simulink library "plant_sim_lib"  (R2022b)
settings: Solver=VariableStepAuto  StartTime=0.0  StopTime=10.0  RelTol=1e-3
libraries: AMK_model_lib x1, battery_model_lib x1, driver_model_lib x1
settings Model: Creator=dr_pa  LastModifiedBy=dr_pa

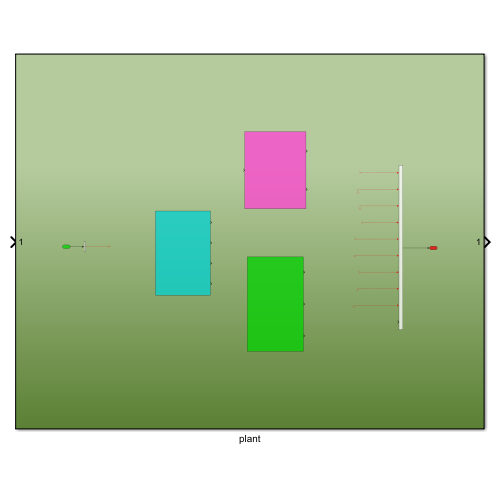
[thumbnail: Simulink's stored preview of the top-level diagram]
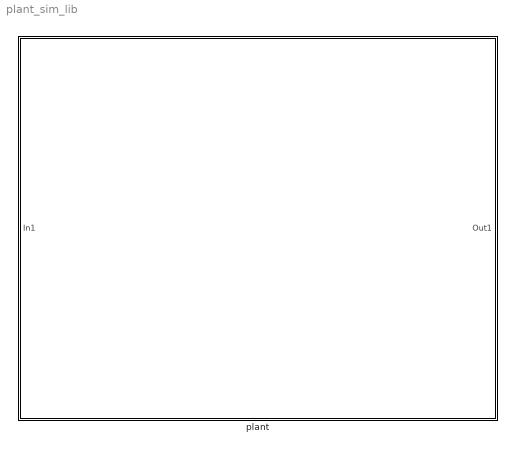
== system plant_sim_lib ==
  plant : Subsystem

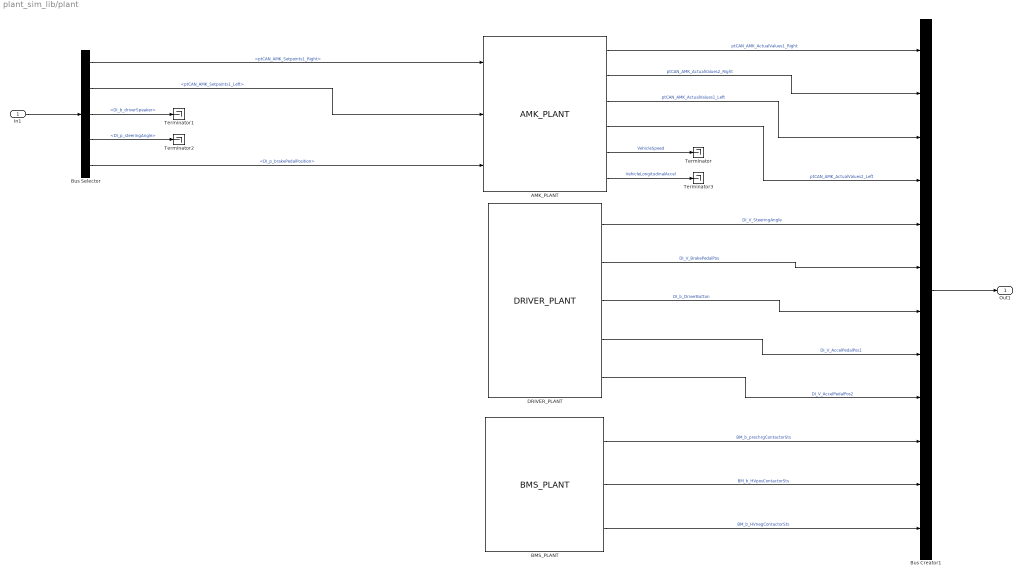
== system plant_sim_lib/plant ==
  In1 : Inport
  AMK_PLANT : AMK_model_lib/AMK_PLANT  SystemSampleTime=-1  VariantActivationTime=update diagram  Latency=0  AutoFrameSizeCalculation=off
  BMS_PLANT : battery_model_lib/BMS_PLANT  SystemSampleTime=-1  VariantActivationTime=update diagram  Latency=0  AutoFrameSizeCalculation=off
  Bus Creator1 : BusCreator  Inputs=12
  Bus Selector : BusSelector  OutputSignals=ptCAN_AMK_Setpoints1_Right,ptCAN_AMK_Setpoints1_Left,DI_b_driverSpeaker,DI_p_steeringAngle,DI_p_brakePedalPosition
  DRIVER_PLANT : driver_model_lib/DRIVER_PLANT  SystemSampleTime=-1  VariantActivationTime=update diagram  Latency=0  AutoFrameSizeCalculation=off
  Terminator{,1..3} (4 alike) : Terminator
  Out1 : Outport
  wires:
  Bus Selector/1 -> AMK_PLANT/1  "<ptCAN_AMK_Setpoints1_Right>"
  DRIVER_PLANT/2 -> Bus Creator1/6  "DI_V_BrakePedalPos"
  AMK_PLANT/2 -> Bus Creator1/2  "ptCAN_AMK_ActualValues2_Right"
  BMS_PLANT/3 -> Bus Creator1/12  "BM_b_HVnegContactorSts"
  AMK_PLANT/4 -> Bus Creator1/4  "ptCAN_AMK_ActualValues2_Left"
  Bus Creator1/1 -> Out1/1
  AMK_PLANT/1 -> Bus Creator1/1  "ptCAN_AMK_ActualValues1_Right"
  DRIVER_PLANT/1 -> Bus Creator1/5  "DI_V_SteeringAngle"
  BMS_PLANT/2 -> Bus Creator1/11  "BM_b_HVposContactorSts"
  DRIVER_PLANT/3 -> Bus Creator1/7  "DI_b_DriverButton"
  DRIVER_PLANT/5 -> Bus Creator1/9  "DI_V_AccelPedalPos2"
  DRIVER_PLANT/4 -> Bus Creator1/8  "DI_V_AccelPedalPos1"
  BMS_PLANT/1 -> Bus Creator1/10  "BM_b_prechrgContactorSts"
  AMK_PLANT/3 -> Bus Creator1/3  "ptCAN_AMK_ActualValues1_Left"
  Bus Selector/2 -> AMK_PLANT/2  "<ptCAN_AMK_Setpoints1_Left>"
  Bus Selector/3 -> Terminator1/1  "<DI_b_driverSpeaker>"
  Bus Selector/4 -> Terminator2/1  "<DI_p_steeringAngle>"
  Bus Selector/5 -> AMK_PLANT/3  "<DI_p_brakePedalPosition>"
  In1/1 -> Bus Selector/1
  AMK_PLANT/5 -> Terminator/1  "VehicleSpeed"
  AMK_PLANT/6 -> Terminator3/1  "VehicleLongitudinalAccel"
